simulink model "MSFartoystyring"  (Simulink 8.4)
settings: Solver=ode45  StartTime=tstart  StopTime=tstop  RelTol=1e-3
values from neighbouring files (symbols this model uses):
  c = 1    [run_task_1_4.m]
  K_d = 2*zeta*Omega_n*(m)-m/T    [run_task_1_4.m]
  K_i = (Omega_n/10)*K_p    [run_task_1_4.m]
  K_p = (m)*Omega_n^2    [run_task_1_4.m]
  psi0 = 0    [run_task_1_4.m]
  r0 = 0    [run_task_1_4.m]
  T = 1/0.006673    (= 149.857635247)    [run_task_1_4.m]    (also in task_1_2.m = x(1))
  tsamp = 10    [run_task_1_4.m]
  v0 = [6.63 0]'    [run_task_1_4.m]
undefined symbols (not defined in the file or in its folder): msfartoystyring
undefined symbols (not defined in the file): p0
settings Model: Creator=christh  LastModifiedBy=Truls  ExtModeAutoUpdateStatusClock=off
settings OptimizationCC: InitFltsAndDblsToZero=on

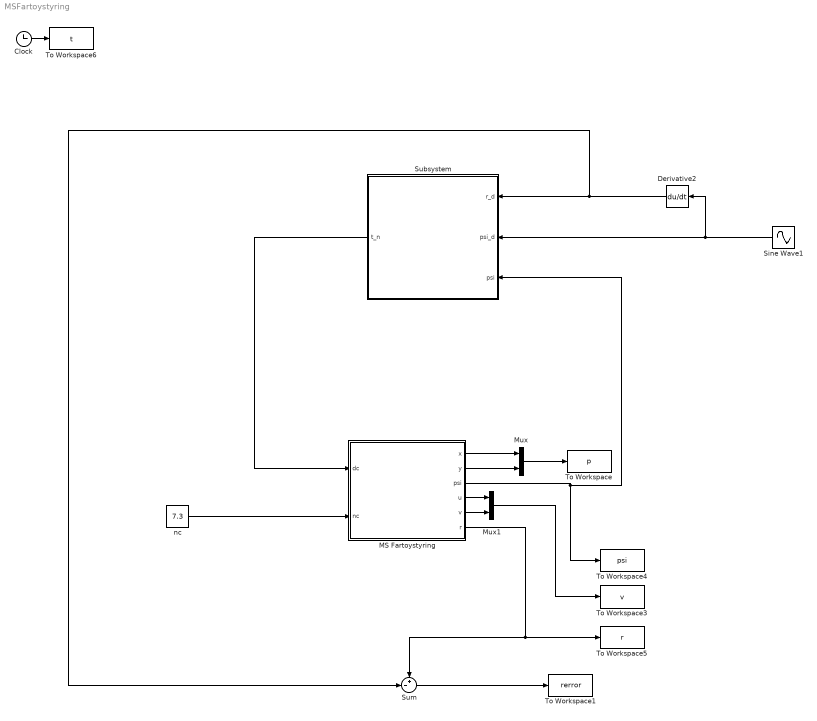
== system MSFartoystyring ==
  Clock : Clock
  Derivative2 : Derivative
  MS Fartoystyring : Subsystem  mask(MS Fartoystyring for Assignment 3 G&C){x0=p0(1), y0=p0(2), u0=v0(1), v0=v0(2), psi0=psi0, r0=r0, c=c}
      mask prompts: x0 "x(t0) (m)"; y0 "y(t0) (m)"; u0 "u(t0) (m/s)"; v0 "v(t0) (m/s)"; psi0 "psi(t0) (rad)"; r0 "r(t0) (rad/s)"; c "current (0 or 1)"
      mask help:
      | Block corresponding to Figure 1 in the assignment text. Gives the response of the ship.
      |
      | The design speed of MS Fartoystyring is u=8.23 m/s.
      |
      | Input:
      | dc: commanded rudder (rad), dmax=25*pi/180
      | nc: commanded shaft speed (rad/s), nmax=85*2*pi/60
      |
      | Output:
      | x: north pos (m)
      | y: east pos (m)
      | u: surge (m/s)
      | v: sway (m/s)
      | psi: heading (rad)
      | r: yaw (rad/s)
      mask Help: Comments, bugs and help requests can be directed to the TA. Email on course website.
  Mux : Mux  Inputs=2
  Mux1 : Mux  Inputs=2
  Sine Wave1 : Sin  Amplitude=-0.3  Frequency=0.008  SampleTime=0
  Subsystem : Subsystem
  Sum : Sum  Inputs=+-|
  To Workspace : ToWorkspace  VariableName=p  SampleTime=tsamp
  To Workspace1 : ToWorkspace  VariableName=rerror  SampleTime=tsamp
  To Workspace3 : ToWorkspace  VariableName=v  SampleTime=tsamp
  To Workspace4 : ToWorkspace  VariableName=psi  SampleTime=tsamp
  To Workspace5 : ToWorkspace  VariableName=r  SampleTime=tsamp
  To Workspace6 : ToWorkspace  VariableName=t  SampleTime=tsamp
  nc : Constant  Value=7.3
  wires:
  Clock/1 -> To Workspace6/1
  MS Fartoystyring/2(y) -> Mux/2
  MS Fartoystyring/4(u) -> Mux1/1
  MS Fartoystyring/5(v) -> Mux1/2
  Mux/1 -> To Workspace/1
  Mux1/1 -> To Workspace3/1
  MS Fartoystyring/3(psi) -> Subsystem/3(psi), To Workspace4/1
  nc/1 -> MS Fartoystyring/2(nc)
  MS Fartoystyring/1(x) -> Mux/1
  MS Fartoystyring/6(r) -> To Workspace5/1, Sum/1
  Derivative2/1 -> Sum/2, Subsystem/1(r_d)
  Sum/1 -> To Workspace1/1
  Subsystem/1(t_n) -> MS Fartoystyring/1(dc)
  Sine Wave1/1 -> Derivative2/1, Subsystem/2(psi_d)

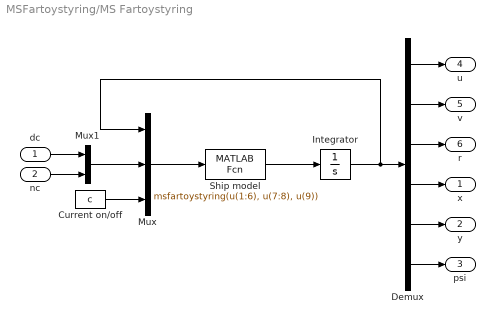
== system MSFartoystyring/MS Fartoystyring ==
  dc : Inport
  nc : Inport  Port=2
  Current on/off : Constant  Value=c
  Demux : Demux  Outputs=6
  Integrator : Integrator  InitialCondition=[u0 v0 r0 x0 y0 psi0]'
  Mux : Mux  Inputs=3
  Mux1 : Mux  Inputs=2
  Ship model : MATLABFcn  MATLABFcn=msfartoystyring(u(1:6), u(7:8), u(9))  OutputDimensions=6
  x : Outport
  y : Outport  Port=2
  psi : Outport  Port=3
  u : Outport  Port=4
  v : Outport  Port=5
  r : Outport  Port=6
  wires:
  Integrator/1 -> Mux/1, Demux/1
  Mux1/1 -> Mux/2
  dc/1 -> Mux1/1
  nc/1 -> Mux1/2
  Demux/1 -> u/1
  Demux/2 -> v/1
  Demux/3 -> r/1
  Demux/4 -> x/1
  Demux/5 -> y/1
  Demux/6 -> psi/1
  Current on/off/1 -> Mux/3
  Ship model/1 -> Integrator/1
  Mux/1 -> Ship model/1

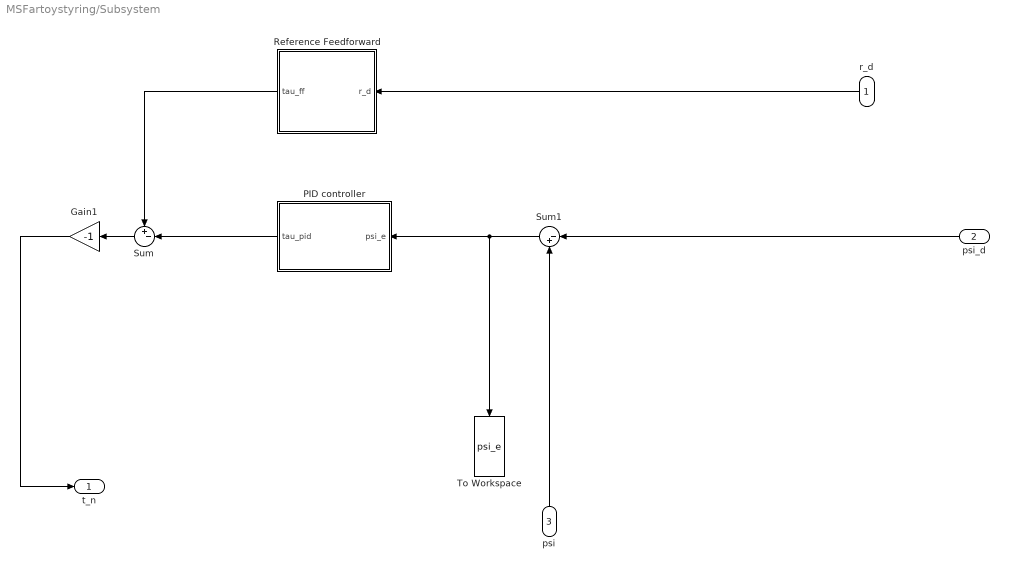
== system MSFartoystyring/Subsystem ==
  r_d : Inport
  psi_d : Inport  Port=2
  psi : Inport  Port=3
  Gain1 : Gain  Gain=-1
  PID controller : Subsystem
  Reference Feedforward : Subsystem
  Sum : Sum  Inputs=+-|
  Sum1 : Sum  Inputs=|-+
  To Workspace : ToWorkspace  VariableName=psi_e  SampleTime=tsamp
  t_n : Outport
  wires:
  psi/1 -> Sum1/2
  Sum/1 -> Gain1/1
  psi_d/1 -> Sum1/1
  Sum1/1 -> PID controller/1(psi_e), To Workspace/1
  PID controller/1(tau_pid) -> Sum/2
  r_d/1 -> Reference Feedforward/1("r_d ")
  Gain1/1 -> t_n/1
  Reference Feedforward/1(tau_ff) -> Sum/1

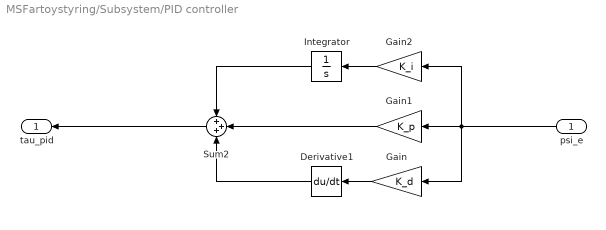
== system MSFartoystyring/Subsystem/PID controller ==
  psi_e : Inport
  Derivative1 : Derivative
  Gain : Gain  Gain=K_d
  Gain1 : Gain  Gain=K_p
  Gain2 : Gain  Gain=K_i
  Integrator : Integrator
  Sum2 : Sum  Inputs=+++
  tau_pid : Outport
  wires:
  Gain1/1 -> Sum2/2
  psi_e/1 -> Gain2/1, Gain/1, Gain1/1
  Integrator/1 -> Sum2/1
  Gain/1 -> Derivative1/1
  Sum2/1 -> tau_pid/1
  Gain2/1 -> Integrator/1
  Derivative1/1 -> Sum2/3

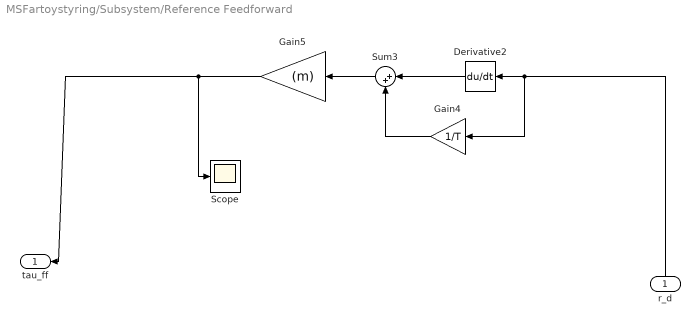
== system MSFartoystyring/Subsystem/Reference Feedforward ==
  "r_d " : Inport
  Derivative2 : Derivative
  Gain4 : Gain  Gain=1/T
  Gain5 : Gain  Gain=(m)
  Scope : Scope
  Sum3 : Sum  Inputs=|++
  tau_ff : Outport
  wires:
  Gain4/1 -> Sum3/2
  Sum3/1 -> Gain5/1
  "r_d "/1 -> Gain4/1, Derivative2/1
  Derivative2/1 -> Sum3/1
  Gain5/1 -> Scope/1, tau_ff/1
